simulink subsystem "VSLIPSL_controller_subsystem"  (R2022b)
settings: Solver=VariableStepAuto  StartTime=0.0  StopTime=10.0  RelTol=1e-3
settings Model: Creator=mmpel  LastModifiedBy=mmpel

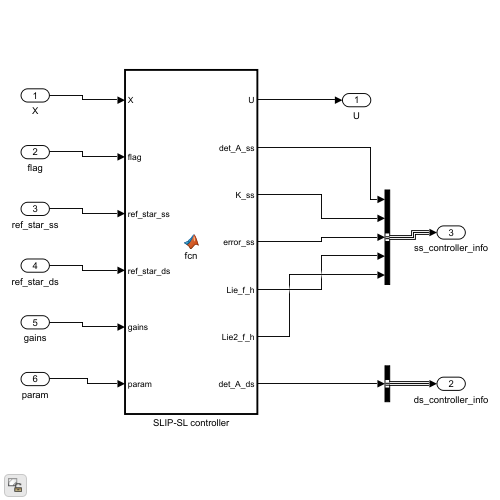
[thumbnail: Simulink's stored preview of the top-level diagram]
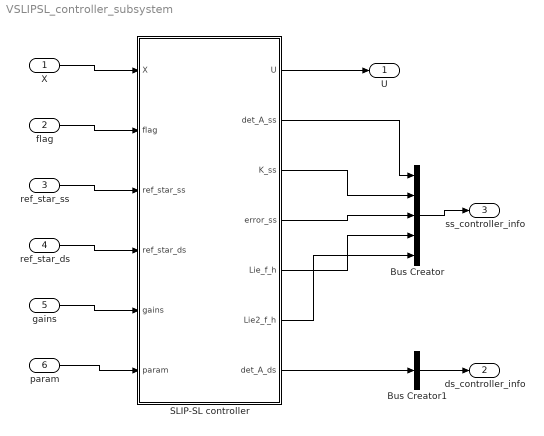
== system VSLIPSL_controller_subsystem ==
  X : Inport
  flag : Inport  Port=2
  ref_star_ss : Inport  Port=3
  ref_star_ds : Inport  Port=4
  gains : Inport  Port=5
  param : Inport  Port=6
  Bus Creator : BusCreator  Inputs=5
  Bus Creator1 : BusCreator  Inputs=1
  SLIP-SL controller : MATLAB Function  TreatAsAtomicUnit=on
  U : Outport
  ds_controller_info : Outport  Port=2
  ss_controller_info : Outport  Port=3
  wires:
  Bus Creator/1 -> ss_controller_info/1
  SLIP-SL controller/6(Lie2_f_h) -> Bus Creator/5
  gains/1 -> SLIP-SL controller/5(gains)
  ref_star_ss/1 -> SLIP-SL controller/3(ref_star_ss)
  SLIP-SL controller/5(Lie_f_h) -> Bus Creator/4
  SLIP-SL controller/4(error_ss) -> Bus Creator/3
  flag/1 -> SLIP-SL controller/2(flag)
  SLIP-SL controller/1(U) -> U/1
  X/1 -> SLIP-SL controller/1(X)
  param/1 -> SLIP-SL controller/6(param)
  SLIP-SL controller/7(det_A_ds) -> Bus Creator1/1
  SLIP-SL controller/2(det_A_ss) -> Bus Creator/1
  SLIP-SL controller/3(K_ss) -> Bus Creator/2
  ref_star_ds/1 -> SLIP-SL controller/4(ref_star_ds)
  Bus Creator1/1 -> ds_controller_info/1

== matlab function VSLIPSL_controller_subsystem/SLIP-SL controller ==
  data: X input; U output; flag input; ref_star_ss input; ref_star_ds input; gains input; param input; det_A_ss output; K_ss output; error_ss output; Lie_f_h output; Lie2_f_h output; det_A_ds output
function [U, det_A_ss, K_ss, error_ss, Lie_f_h, Lie2_f_h, det_A_ds] = fcn(X, flag, ref_star_ss, ref_star_ds, gains, param)

% ----------- parameters ----------------------
L0_ss = param(1); % [m]
k0_ss = param(2); % nominal leg stiffness [N/m]
m_M = param(3); % hip mass [kg]
m_swLeg = param(4); % [kg]
m_swFoot = param(5); % [kg]
I_swLeg = param(6); %
I_swFoot = param(7); %
L_thigh = param(8); % [m]
k_swFoot = param(9); %
k_swLeg = param(10); %
theta0 = param(11); %[rad]
r0 = param(12); % [m]
gravi = param(13); % gravitational acc

L0_ds = param(14); % [m] free length of the springs in the DS
k0_ds = param(15); % [N/m] stiffness of the springs in the DS

% ----------- flags ----------------------
f_stance = flag(1); % indicates which stance phase it is
foot = flag(2); % location of the stance foot
foot_prev = flag(3) - foot; % previous location of the stance foot
x_CoM_TD = flag(4) - foot; % x_CoM @TD
x_CoM_LO = flag(5); % x_CoM @LO
flag_ref_ob = flag(6); % raised if ref. state var. starts out of bounds at stage trans.

% ----------- states ----------------------
x_M = X(1) - foot; % x position of main mass in SS
y_M = X(2); % z position of main mass in SS
theta = X(3); % angle of the swing leg when in SS
r = X(4); % distance of the foot from the knee on SS
x_CoM = X(5) - foot; % x position of the CoM
y_CoM = X(6);

dx_M = X(7); % x velocity of main mass in SS
dy_M = X(8); % z velocity of main mass in SS
dtheta = X(9);
dr = X(10);
dx_CoM = X(11);
dy_CoM = X(12);

q = [x_M; y_M; theta; r; x_CoM; y_CoM];
dq = [dx_M; dy_M; dtheta; dr; dx_CoM; dy_CoM];

%---------- controller -----------------------------

% SS inputs
u1 = 0; % input for stance leg spring
u2 = 0; % input for swing leg torsional spring
u3 = 0; % input for swing foot spring
% DS inputs
u4 = 0; % input for stance leg spring
u5 = 0; % input for swing leg spring

% for debugging
det_A_ss = NaN;
K_ss = [NaN; NaN; NaN];
error_ss = [NaN; NaN; NaN];
Lie_f_h = [NaN; NaN; NaN];
Lie2_f_h = [NaN; NaN; NaN];

det_A_ds = 0;

x_CoM_star_ss = ref_star_ss(:,11);
x_CoM_star_ds = ref_star_ds(:,1);

%%

if f_stance == 1
    % if the system is in single stance phase

    % Calculating the phase variable x_CoM
    x_swLeg = x_M + (L_thigh/2)*cos(theta);
    x_swFoot = x_M + (L_thigh + r)*cos(theta);
    x_CoM = (m_M*x_M + m_swLeg*x_swLeg + m_swFoot*x_swFoot)/(m_M + m_swLeg + m_swFoot);

    if x_CoM_star_ss(1) <= x_CoM && x_CoM <= x_CoM_star_ss(end)

        % testing function implementation
        X_slipsl_ss = [x_M; y_M; theta; r; dx_M; dy_M; dtheta; dr];
        [U_ss, det_A_ss, K_ss, error_ss, Lie_f_h, Lie2_f_h] = VSLIPSL_controller_SS( ...
            x_CoM, X_slipsl_ss, ref_star_ss, param, gains);

        u1 = U_ss(1);
        u2 = U_ss(2);
        u3 = U_ss(3);

    end

else
    % if the system is in double stance phace

    if x_CoM_star_ds(1) <= x_CoM && x_CoM <= x_CoM_star_ds(end)
    % if x_CoM <= x_CoM_star_ds(end)
        
        X_slipsl_ds = [x_CoM; y_CoM; dx_CoM; dy_CoM];
        [U_ds_test, det_A_ds] = VSLIPSL_controller_DS( ...
                x_CoM, X_slipsl_ds, flag, ref_star_ds, param, gains);

        u4 = U_ds_test(1);
        u5 = U_ds_test(2);
    end

end

U = [u1; u2; u3; u4; u5];

% clipped = max(min(x, upper), lower);
var_stiff_bound_cst = 0.5;
upper = (1 + var_stiff_bound_cst);
lower = (var_stiff_bound_cst - 1);
U = [
    max(min(u1, k0_ss*upper), k0_ss*lower);
    max(min(u2, k_swLeg*upper), k_swLeg*lower);
    max(min(u3, k_swFoot*upper), k_swFoot*lower);
    max(min(u4, k0_ds*upper), k0_ds*lower);
    max(min(u5, k0_ds*upper), k0_ds*lower)];
